simulink model "test_nlmpcMultistage_withIntegralControl"  (R2024b)
settings: Solver=VariableStepAuto  StartTime=0.0  StopTime=20  RelTol=1e-3
values from neighbouring files (symbols this model uses):
  msobj = nlmpcMultistage(predHorizon, nx_extended, nu)    [NonlinearSystemControl_withKoopman_and_nlmpcMultistage.m]
  predHorizon = pvstage(2)    [MyNMPC.m]    (also in NonlinearSystemControl_withKoopman_and_nlmpcMultistage.m = 10)
  pvcost = [current_ref; predHorizon; Q; R; S; Qi]    [NonlinearSystemControl_withKoopman_and_nlmpcMultistage.m]
  Q = pvstage(3)    [MyNMPC.m]    (also in NonlinearSystemControl_withKoopman_and_nlmpcMultistage.m = 10)
  Qi = pvstage(6)    [MyNMPC.m]    (also in NonlinearSystemControl_withKoopman_and_nlmpcMultistage.m = 1)
  R = pvstage(4)    [MyNMPC.m]    (also in NonlinearSystemControl_withKoopman_and_nlmpcMultistage.m = 0.1)
  S = pvstage(5)    [MyNMPC.m]    (also in NonlinearSystemControl_withKoopman_and_nlmpcMultistage.m = 20)
undefined symbols (not defined in the file or in its folder): model, params
settings Model: Creator=fnae  LastModifiedBy=fnae
settings DebuggingCC: UnconnectedInputMsg=warning  UnconnectedOutputMsg=warning  UnconnectedLineMsg=warning
settings ModelReferenceCC: EnableRefExpFcnMdlSchedulingChecks=on
settings RTWCC: GPUComputeCapability=3.5  DLArmComputeVersion=19.05

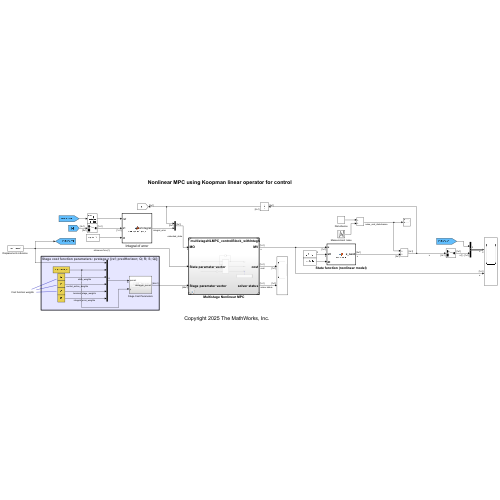
[thumbnail: Simulink's stored preview of the top-level diagram]
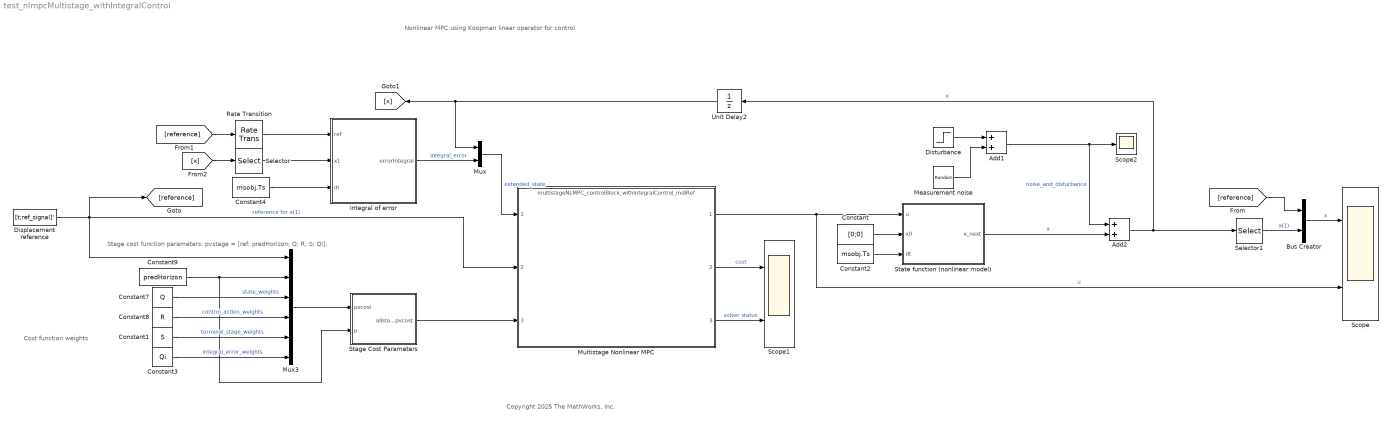
== system test_nlmpcMultistage_withIntegralControl ==
  note: Nonlinear MPC using Koopman linear operator for control
  note: Cost function weights
  note: Copyright 2025 The MathWorks, Inc.
  note: Stage cost function parameters: pvstage = [ref; predHorizon; Q; R; S; Qi];
  Add1 : Sum
  Add2 : Sum
  Bus Creator : BusCreator  Inputs=2
  Constant : Constant  Value=[0;0]
  Constant1 : Constant  Value=S
  Constant2 : Constant  Value=msobj.Ts
  Constant3 : Constant  Value=Qi
  Constant4 : Constant  Value=msobj.Ts
  Constant7 : Constant  Value=Q
  Constant8 : Constant  Value=R
  Constant9 : Constant  Value=predHorizon
  "Displacement reference " : FromWorkspace  VariableName=[t;ref_signal]'
  Disturbance : Step  Time=5  After=0.1  SampleTime=0
  Integral of error : MATLAB Function  TreatAsAtomicUnit=on
  Measurement noise : UniformRandomNumber  Minimum=-0.03  Maximum=0.03  SampleTime=msobj.Ts
  Multistage Nonlinear MPC : ModelReference  ModelNameDialog=multistageNLMPC_controlBlock_withIntegralControl_mdlRef.slx  SimulationMode=Normal  ModelReferenceVersion=3.9
  Mux : Mux  Inputs=2
  Mux3 : Mux  Inputs=6
  Rate Transition : RateTransition  OutPortSampleTime=msobj.Ts
  Scope : Scope  NumInputPorts=2
  Scope1 : Scope  NumInputPorts=2
  Scope2 : Scope
  Selector : Selector  InputPortWidth=nx  IndexOptions=Index vector (dialog)  Indices=1  OutputSizes=1
  Selector1 : Selector  InputPortWidth=nx  IndexOptions=Index vector (dialog)  Indices=1  OutputSizes=1
  Stage Cost Parameters : Subsystem
  State function (nonlinear model) : MATLAB Function  TreatAsAtomicUnit=on
  Unit Delay2 : UnitDelay  InitialCondition=[0;0]  SampleTime=msobj.Ts  HasFrameUpgradeWarning=on
  wires:
  Unit Delay2/1 -> Mux/1, [x]
  Add2/1 -> Unit Delay2/1, Selector1/1  "x"
  Disturbance/1 -> Add1/1
  Bus Creator/1 -> Scope/1  "x"
  Constant9/1 -> Stage Cost Parameters/2(p), Mux3/2
  Mux3/1 -> Stage Cost Parameters/1(pvcost)
  [reference] -> Bus Creator/1
  Multistage Nonlinear MPC/2 -> Scope1/1  "cost"
  Multistage Nonlinear MPC/3 -> Scope1/2  "solver status"
  Constant7/1 -> Mux3/3  "state_weights"
  Constant8/1 -> Mux3/4  "control_action_weights"
  Constant1/1 -> Mux3/5  "terminal_stage_weights"
  Multistage Nonlinear MPC/1 -> Scope/2, State function (nonlinear model)/1(u)  "u"
  Constant3/1 -> Mux3/6  "integral_error_weights"
  Mux/1 -> Multistage Nonlinear MPC/1  "extended_state"
  [x] -> Selector/1
  Stage Cost Parameters/1(allstages_pvcost) -> Multistage Nonlinear MPC/3
  Integral of error/1(errorIntegral) -> Mux/2  "integral_error"
  "Displacement reference "/1 -> Mux3/1, Multistage Nonlinear MPC/2, [reference]  "reference for x(1)"
  Selector/1 -> Integral of error/2(x1)
  [reference] -> Rate Transition/1
  Constant/1 -> State function (nonlinear model)/2(x0)
  Constant2/1 -> State function (nonlinear model)/3(dt)
  State function (nonlinear model)/1(x_next) -> Add2/2  "x"
  Constant4/1 -> Integral of error/3(dt)
  Rate Transition/1 -> Integral of error/1(ref)
  Selector1/1 -> Bus Creator/2  "x(1)"
  Measurement noise/1 -> Add1/2
  Add1/1 -> Add2/1, Scope2/1  "noise_and_disturbance"

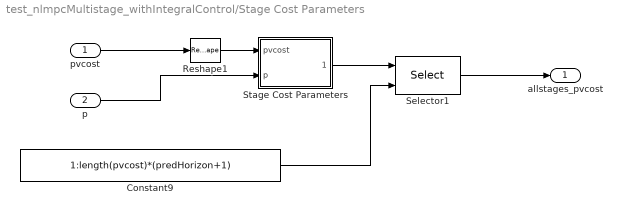
== system test_nlmpcMultistage_withIntegralControl/Stage Cost Parameters ==
  pvcost : Inport
  p : Inport  Port=2
  Constant9 : Constant  Value=1:length(pvcost)*(predHorizon+1)
  Reshape1 : Reshape  OutputDimensionality=Column vector (2-D)
  Selector1 : Selector  InputPortWidth=length(pvcost)*(predHorizon+1)  IndexOptions=Index vector (port)  Indices=1:length(repmat(params,model.N,1))  OutputSizes=1
  Stage Cost Parameters : MATLAB Function  TreatAsAtomicUnit=on
  allstages_pvcost : Outport
  wires:
  Selector1/1 -> allstages_pvcost/1
  pvcost/1 -> Reshape1/1
  Reshape1/1 -> Stage Cost Parameters/1(pvcost)
  Stage Cost Parameters/1(stageCost) -> Selector1/1
  Constant9/1 -> Selector1/2
  p/1 -> Stage Cost Parameters/2(p)

== matlab function test_nlmpcMultistage_withIntegralControl/Integral of error ==
  data: ref input; errorIntegral output; x1 input; dt input
function errorIntegral = integral_of_error(ref, x1, dt)
%#codegen

persistent e_i

if isempty(e_i)
    e_i = 0;
end

% Update integral error
e_i = e_i + dt*(ref - x1);  

errorIntegral = e_i;

== matlab function test_nlmpcMultistage_withIntegralControl/State function (nonlinear model) ==
  data: u input; x0 input; x_next output; dt input
function x_next = stateFcn(u, x0, dt)
%#codegen

persistent x

if isempty(x)
    x = x0;
end

% Define state evolution function
dxdt = [(x(2) + 0.5*u); -sin(x(1)) - 0.2*x(2) + u];

% Euler integration for next state
x = x + dt*dxdt;

x_next = x;

end

== matlab function test_nlmpcMultistage_withIntegralControl/Stage Cost Parameters/Stage Cost Parameters ==
  settings: updateMethod=DISCRETE  sampleTime=msobj.Ts
  data: pvcost input; stageCost output size=[length(pvcost)*(predHorizon+1),1]; p input
function stageCost = fcn(pvcost,p)

stageCost = repmat(pvcost, p+1, 1);
